simulink model "solarrrrr"  (R2015a)
settings: Solver=ode23t  StartTime=0.0  StopTime=1  RelTol=1e-3
undefined symbols (not defined in the file): Ion, Lithium, sigbuilder_block
libraries: powerlib x11, simulink x3, electricdrivelib x1, re_lib x1
settings Model: Creator=Viren S. Ram  LastModifiedBy=Viren S. Ram

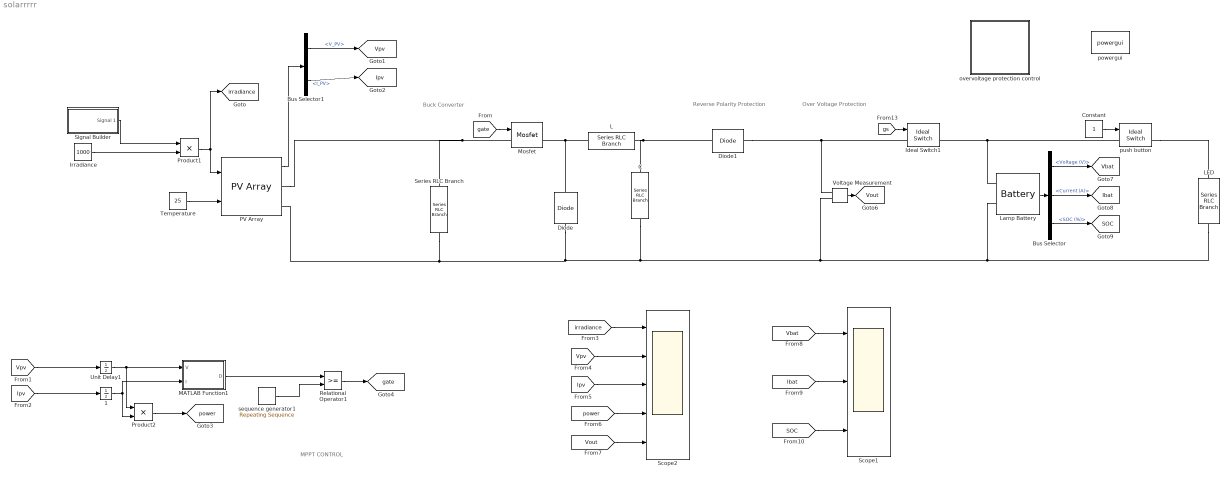
== system solarrrrr ==
  note: Over Voltage Protection
  note: Reverse Polarity
      |         Protection
  note: MPPT CONTROL
  note: Buck Converter
  " 1" : UnitDelay  SampleTime=1e-4
  Bus Selector : BusSelector  OutputSignals=Voltage (V),Current (A),SOC (%)
  Bus Selector1 : BusSelector  OutputSignals=V_PV,I_PV
  C : powerlib/Elements/Series RLC Branch  LConnTagsString=__new0  RConnTagsString=__new0  BranchType=C  Resistance=0.0001  Inductance=0.783e-3  SetiL0=off  InitialCurrent=0  Capacitance=600e-6  Setx0=off  InitialVoltage=0  Measurements=None
  Constant : Constant
  Diode : powerlib/Power Electronics/Diode  Ron=0.001  Lon=0  Vf=0.8  IC=0  UseSnubber=off  Rs=500  Cs=250e-9  Measurements=off
  Diode1 : powerlib/Power Electronics/Diode  Ron=0.001  Lon=0  Vf=0.8  IC=0  UseSnubber=off  Rs=500  Cs=250e-9  Measurements=off
  Ideal Switch1 : powerlib/Power Electronics/Ideal Switch  Ron=0.001  Lon=0  IC=1  Rs=1e5  Cs=inf  Measurements=on
  Irradiance : Constant  Value=1000
  L : powerlib/Elements/Series RLC Branch  LConnTagsString=__new0  RConnTagsString=__new0  BranchType=L  Resistance=0.0001  Inductance=0.783e-3  SetiL0=off  InitialCurrent=0  Capacitance=1000e-6  Setx0=off  InitialVoltage=0  Measurements=None
  "LED " : powerlib/Elements/Series RLC Branch  LConnTagsString=__new0  RConnTagsString=__new0  BranchType=R  Resistance=10  Inductance=1e-3  SetiL0=off  InitialCurrent=0  Capacitance=1e-6  Setx0=off  InitialVoltage=0  Measurements=None
  Lamp Battery : electricdrivelib/Extra Sources/Battery  BatType=Lithium-Ion  ShowDetailedParameters=off  NomV=12  NomQ=100  SOC=45  PresetModel=on  MaxQ=100  FullV=13.9678  Dis_rate=43.4783  R=0.0012  Normal_OP=90.4348  expZone="[12.9646      4.91304]"  current=[6.5 13 32.5]  Units=Time  Batt_Tr=1e-6
  MATLAB Function1 : MATLAB Function  TreatAsAtomicUnit=on
  Mosfet : powerlib/Power Electronics/Mosfet  Ron=0.1  Lon=0  Rd=0.01  Vfd=0  IC=0  Rs=1e5  Cs=inf  Measurements=on
  PV Array : re_lib/Solar/PV Array  Npar=1  Nser=1  PlotType=array @ 25 deg.C & specified irradiances  S_vec="[ 1000  500  100 ]"  Temp_C_vec="[ 45 25  ]"  ModuleName=1Soltech 1STH-215-P  PlotWhenSelected=off  Pm=213.15  Ncell=60  Voc=36.3  Isc=7.84  Vm=29  Im=7.35  beta_Voc_pc=-0.36099  alpha_Isc_pc=0.102  beta_Voc=-0.13104  alpha_Isc=0.007997  IL=7.8649  I0=2.9259e-10  nI=0.98117  Rsh=313.3991  Rs=0.39383  BAL=on  Tc=1e-6  Tfilter=5e-5
  Product1 : Product
  Product2 : Product
  Relational Operator1 : RelationalOperator  OutDataTypeStr=boolean
  Scope1 : Scope  NumInputPorts=3
      settings: TimeRange=1  YMin=12.9~-500~45  YMax=13.5~0~45.0018  SaveName=soc
  Scope2 : Scope  NumInputPorts=5
      settings: TimeRange=2  YMin=45~-5~-5~-5~-5  YMax=45.0065~5~5~5~5  SaveName=soc1
  Series RLC Branch : powerlib/Elements/Series RLC Branch  LConnTagsString=__new0  RConnTagsString=__new0  BranchType=RC  Resistance=0.0001  Inductance=1e-3  SetiL0=off  InitialCurrent=0  Capacitance=1000e-6  Setx0=off  InitialVoltage=0  Measurements=None
  Signal Builder : Subsystem  Tag=STV Subsys  LoadFcn=sigbuilder_block('load');  StartFcn=sigbuilder_block('start');  StopFcn=sigbuilder_block('stop');  ClipboardFcn=sigbuilder_block('clipboard');  mask(Sigbuilder block){}
      mask help: Simulink:masks:SigbuilderBlock_MD
      mask init:
      | if ~strcmp(get_param(bdroot(gcbh),'SimulationStatus'),'stopped') tuvar = sigbuilder_block('maskInit'); end
      settings: CopyFcn=sigbuilder_block('copy');  DeleteFcn=sigbuilder_block('delete');  ModelCloseFcn=sigbuilder_block('modelClose');  PreSaveFcn=sigbuilder_block('preSave');  PauseFcn=sigbuilder_block('pause');  ContinueFcn=sigbuilder_block('continue');  NameChangeFcn=sigbuilder_block('namechange');  OpenFcn=sigbuilder_block('open',[437.6 199.2 550.4 400 ]);  CloseFcn=sigbuilder_block('close');
      mask Display: plot(0, 0, 100, 100,[2, 2, 32, 32, 2], [68, 8, 8, 68, 68],[32, 2], [38, 38], [32, 19, 2],[53, 60, 44], [32, 17, 17, 2],[16, 16, 31, 31]);txt = getActiveGroup(gcbh);text(2, 100, txt,'verticalAlignment', 'top');
  Temperature : Constant  Value=25
  Unit Delay1 : UnitDelay  SampleTime=1e-4
  Voltage Measurement : powerlib/Measurements/Voltage Measurement  PhasorSimulation=off  OutputType=Complex  PSBequivalent=0
  "overvoltage protection control " : Subsystem
  powergui : powerlib/powergui  Priority=1  SimulationMode=Discrete  SolverType=Tustin/Backward Euler (TBE)  SampleTime=1e-6  frequency=60  SPID=off  DisableSnubberDevices=off  DisableRonSwitches=off  DisableVfSwitches=off  SwTol=0  DisplayEquations=off  Interpol=off  methode=off  Ts=100  FunctionMessages=off  echomessages=off  HookPort=off  EnableUseOfTLC=off  x0status=blocks  frequencyindice=0  Pbase=100e6  ErrMax=1e-4  Iterations=50  UnitsV=kV  UnitsW=MW  buscounter=0  RestoreLinks=warning  ResistiveCurrentMeasurement=off  Frange=[0:2:500]  Ylog=off  Xlog=on  ShowGrid=off  save=off  variable=ZData  structure=0  ZoomFFT=off  StartTime=0.0  cycles=1  DisplayStyle=1  fundamental=60  FreqAxis=off  MaxFrequency=1000  frequencyindicesteady=1  RmsSteady=1  display=off
  push button : powerlib/Power Electronics/Ideal Switch  Ron=0.001  Lon=0  IC=0  Rs=1e5  Cs=inf  Measurements=on
  sequence generator1 : simulink/Sources/Repeating Sequence  rep_seq_t=[0 0.0002]  rep_seq_y=[0 1]
  tag scope: Ibat=global, Ipv=global, SOC=global, Vbat=global, Vout=global, Vpv=global, gate=global, irradiance=global, power=global
  wires:
  Temperature/1 -> PV Array/2
  Lamp Battery/1 -> Bus Selector/1
  PV Array/1 -> Bus Selector1/1
  Signal Builder/1(Signal 1) -> Product1/1
  Irradiance/1 -> Product1/2
  Product1/1 -> [irradiance], PV Array/1
  [gate] -> Mosfet/1
  [Vpv] -> Unit Delay1/1
  [Ipv] -> " 1"/1
  Unit Delay1/1 -> MATLAB Function1/1(V), Product2/1
  " 1"/1 -> MATLAB Function1/2(I), Product2/2
  Product2/1 -> [power]
  MATLAB Function1/1(D) -> Relational Operator1/1
  sequence generator1/1 -> Relational Operator1/2
  Relational Operator1/1 -> [gate]
  Bus Selector1/1 -> [Vpv]  "<V_PV>"
  Bus Selector1/2 -> [Ipv]  "<I_PV>"
  Voltage Measurement/1 -> [Vout]
  [irradiance] -> Scope2/1
  [Vpv] -> Scope2/2
  [Ipv] -> Scope2/3
  [power] -> Scope2/4
  [Vout] -> Scope2/5
  Bus Selector/3 -> [SOC]  "<SOC (%)>"
  Bus Selector/2 -> [Ibat]  "<Current (A)>"
  Bus Selector/1 -> [Vbat]  "<Voltage (V)>"
  [Vbat] -> Scope1/1
  [Ibat] -> Scope1/2
  [SOC] -> Scope1/3
  Constant/1 -> push button/1
  [gs] -> Ideal Switch1/1
  connections:
  PV Array/RConn1 -- Mosfet/LConn1 -- Series RLC Branch/LConn1
  Series RLC Branch/RConn1 -- "LED "/RConn1 -- Lamp Battery/LConn2 -- Voltage Measurement/LConn2 -- C/RConn1 -- Diode/LConn1 -- PV Array/RConn2
  L/RConn1 -- Diode/RConn1 -- Mosfet/RConn1
  Diode1/RConn1 -- Ideal Switch1/LConn1 -- Voltage Measurement/LConn1
  C/LConn1 -- Diode1/LConn1 -- L/LConn1
  Ideal Switch1/RConn1 -- Lamp Battery/LConn1 -- push button/LConn1
  push button/RConn1 -- "LED "/LConn1

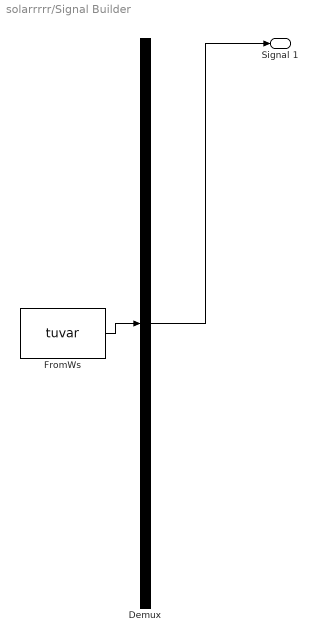
== system solarrrrr/Signal Builder ==
  Demux : Demux  Tag=STV Demux  Outputs=1
  FromWs : FromWorkspace  Tag=STV FromWs  VariableName=tuvar  SampleTime=0
      SigBuilderData=|
      | common.afterFinalStr = 'Extrapolate'
      | common.sampleTime = 0
      | dataSet.timeRange = [0 2]
      | dataSet.name = 'Group 1'
      | sbobj.Groups.Name = 'Group 1'
      | sbobj.Groups.Signals.Name = 'Signal 1'
      | sbobj.Groups.Signals.XData = [0 0.53 0.53 0.95 0.95 1.4 1.4 2]
      | sbobj.Groups.Signals.YData = [1 0.998 0.902 0.9 0.798 0.794 0.96 0.958]
      | sbobj.Groups.TimeRange = [0 2]
  Signal 1 : Outport  Tag=STV Outport
  wires:
  Demux/1 -> Signal 1/1
  FromWs/1 -> Demux/1

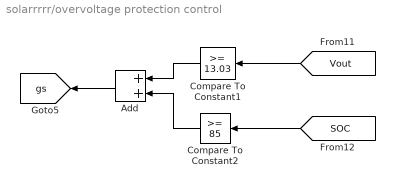
== system solarrrrr/overvoltage protection control  ==
  Add : Sum
  Compare To Constant1 : simulink/Logic and Bit Operations/Compare To Constant  relop=>=  const=13.03  OutDataTypeStr=boolean
  Compare To Constant2 : simulink/Logic and Bit Operations/Compare To Constant  relop=>=  const=85  OutDataTypeStr=boolean
  tag scope: gs=global
  wires:
  Compare To Constant1/1 -> Add/1
  [SOC] -> Compare To Constant2/1
  [Vout] -> Compare To Constant1/1
  Add/1 -> [gs]
  Compare To Constant2/1 -> Add/2

== matlab function solarrrrr/MATLAB Function1 ==
  data: V input; D output; I input
function D = DutyRatio(V, I)

Dmax = 0.95;
Dmin = 0;
Dinit = 0.95;
deltaD = 0.0001;
persistent Vold Pold Dold;

dataType = 'double';

if isempty(Vold)
    Vold = 0;
    Pold = 0;
    Dold = Dinit;
end

P=V*I;
dV = V-Vold;
dP = P-Pold;

if dP ~= 0
    if dP<0
        if dV<0
            D=Dold-deltaD;
        else
            D=Dold+deltaD;
        end
    else
        if dV<0
            D = Dold + deltaD;
        else
            D = Dold - deltaD;
        end
    end
else D=Dold;
end

if D>=Dmax || D <=Dmin
    D = Dold;
end

Dold=D;
Vold=V;
Pold=P;
